simulink model "projectile_motion_horizontal_distance"  (R2021a)
settings: Solver=VariableStepAuto  StartTime=0.0  StopTime=10.0  RelTol=1e-3
InitFcn:
  | theta=30
  | g=9.8
  | v0 =10
libraries: simulink_extras x2
settings Model: Creator=DELL  LastModifiedBy=DELL

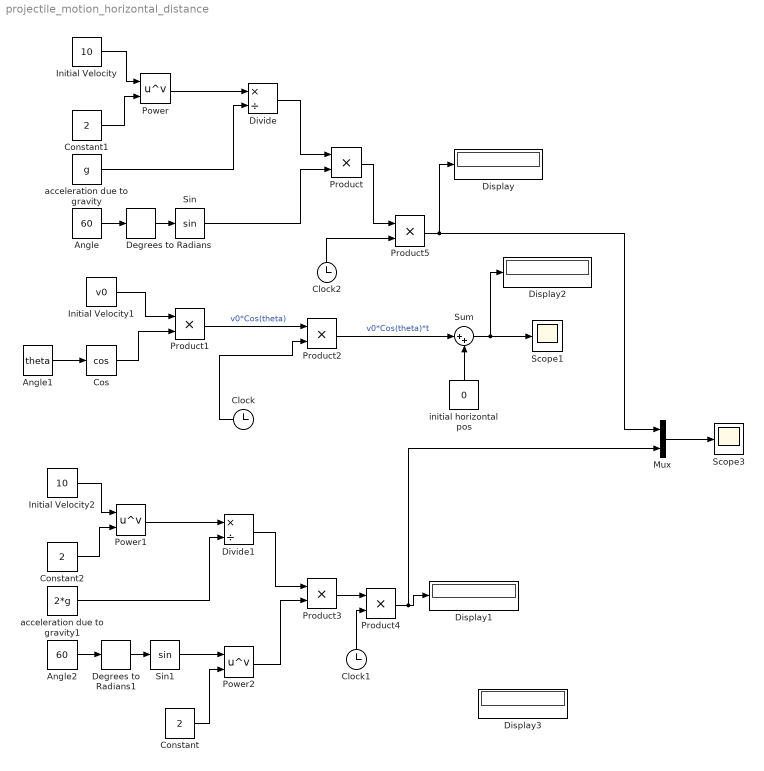
== system projectile_motion_horizontal_distance ==
  Angle : Constant  Value=60
  Angle1 : Constant  Value=theta
  Angle2 : Constant  Value=60
  Clock : Clock
  Clock1 : Clock
  Clock2 : Clock
  Constant : Constant  Value=2
  Constant1 : Constant  Value=2
  Constant2 : Constant  Value=2
  Cos : Trigonometry  Operator=cos
  Degrees to Radians : simulink_extras/Transformations/Degrees to Radians
  Degrees to Radians1 : simulink_extras/Transformations/Degrees to Radians
  Display{,1..3} (4 alike) : Display
  Divide : Product  Inputs=*/
  Divide1 : Product  Inputs=*/
  Initial Velocity : Constant  Value=10
  Initial Velocity1 : Constant  Value=v0
  Initial Velocity2 : Constant  Value=10
  Mux : Mux  Inputs=2
  Power : Math  Operator=pow  SaturateOnIntegerOverflow=on
  Power1 : Math  Operator=pow  SaturateOnIntegerOverflow=on
  Power2 : Math  Operator=pow  SaturateOnIntegerOverflow=on
  Product{,1..5} (6 alike) : Product
  Scope1 : Scope
  Scope3 : Scope
  Sin : Trigonometry
  Sin1 : Trigonometry
  Sum : Sum  Inputs=|++
  acceleration due to gravity : Constant  Value=g
  acceleration due to gravity1 : Constant  Value=2*g
  initial horizontal pos : Constant  Value=0
  wires:
  Initial Velocity/1 -> Power/1
  Constant1/1 -> Power/2
  acceleration due to gravity/1 -> Divide/2
  Power/1 -> Divide/1
  Angle1/1 -> Cos/1
  Cos/1 -> Product1/2
  Initial Velocity1/1 -> Product1/1
  Product1/1 -> Product2/1  "v0*Cos(theta)"
  Clock/1 -> Product2/2
  Product2/1 -> Sum/1  "v0*Cos(theta)*t"
  initial horizontal pos/1 -> Sum/2
  Sum/1 -> Display2/1, Scope1/1
  Degrees to Radians/1 -> Sin/1
  Angle/1 -> Degrees to Radians/1
  Sin/1 -> Product/2
  Divide/1 -> Product/1
  Product/1 -> Product5/1
  Angle2/1 -> Degrees to Radians1/1
  Divide1/1 -> Product3/1
  Degrees to Radians1/1 -> Sin1/1
  Initial Velocity2/1 -> Power1/1
  Power1/1 -> Divide1/1
  Constant2/1 -> Power1/2
  acceleration due to gravity1/1 -> Divide1/2
  Sin1/1 -> Power2/1
  Constant/1 -> Power2/2
  Power2/1 -> Product3/2
  Mux/1 -> Scope3/1
  Product3/1 -> Product4/1
  Product4/1 -> Mux/2, Display1/1
  Clock1/1 -> Product4/2
  Clock2/1 -> Product5/2
  Product5/1 -> Display/1, Mux/1
